simulink model "untitled1"  (R2021a)
settings: Solver=VariableStepAuto  StartTime=0.0  StopTime=10.0  RelTol=1e-3
undefined symbols (not defined in the file): b, K1, K12, M1, M2
settings Model: Creator=AVM  LastModifiedBy=AVM

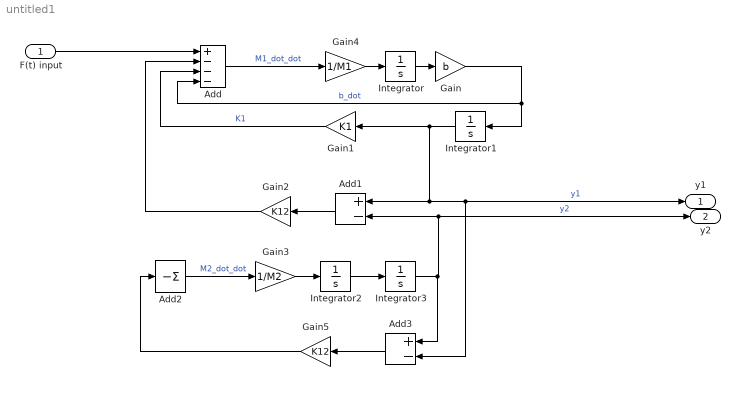
== system untitled1 ==
  F(t) input : Inport
  Add : Sum  Inputs=+---
  Add1 : Sum  Inputs=+-
  Add2 : Sum  Inputs=-
  Add3 : Sum  Inputs=+-
  Gain : Gain  Gain=b
  Gain1 : Gain  Gain=K1
  Gain2 : Gain  Gain=K12
  Gain3 : Gain  Gain=1/M2
  Gain4 : Gain  Gain=1/M1
  Gain5 : Gain  Gain=K12
  Integrator{,1..3} (4 alike) : Integrator
  y1 : Outport
  y2 : Outport  Port=2
  wires:
  Gain3/1 -> Integrator2/1
  F(t) input/1 -> Add/1
  Gain4/1 -> Integrator/1
  Integrator/1 -> Gain/1
  Integrator2/1 -> Integrator3/1
  Integrator3/1 -> Add3/1, y2/1, Add1/2  "y2"
  Add3/1 -> Gain5/1
  Add1/1 -> Gain2/1
  Gain2/1 -> Add/2
  Gain1/1 -> Add/3  "K1"
  Gain5/1 -> Add2/1
  Gain/1 -> Add/4, Integrator1/1  "b_dot"
  Add2/1 -> Gain3/1  "M2_dot_dot"
  Integrator1/1 -> y1/1, Add3/2, Add1/1, Gain1/1  "y1"
  Add/1 -> Gain4/1  "M1_dot_dot"
